simulink model "TST_EngDem_TrqLimCoord"  (R2016b)
settings: Solver=FixedStepDiscrete  StartTime=0.0  StopTime=0  FixedStep=sampleTime  RelTol=1e-3
values from neighbouring files (symbols this model uses):
  testCase = 1    [initTST_EngDem_TrqLimCoord_001.m]    (also in initTST_EngDem_TrqLimCoord_002.m = 2; initTST_EngDem_TrqLimCoord_003.m = 3; initTST_EngDem_TrqLimCoord_004.m = 4)
libraries: simulink x33, UnitTest_Lib x28
(part 1 of 2)
settings Model: Creator=zhengjinyan  LastModifiedBy=zhengjinyan
settings DebuggingCC: SignalRangeChecking=error

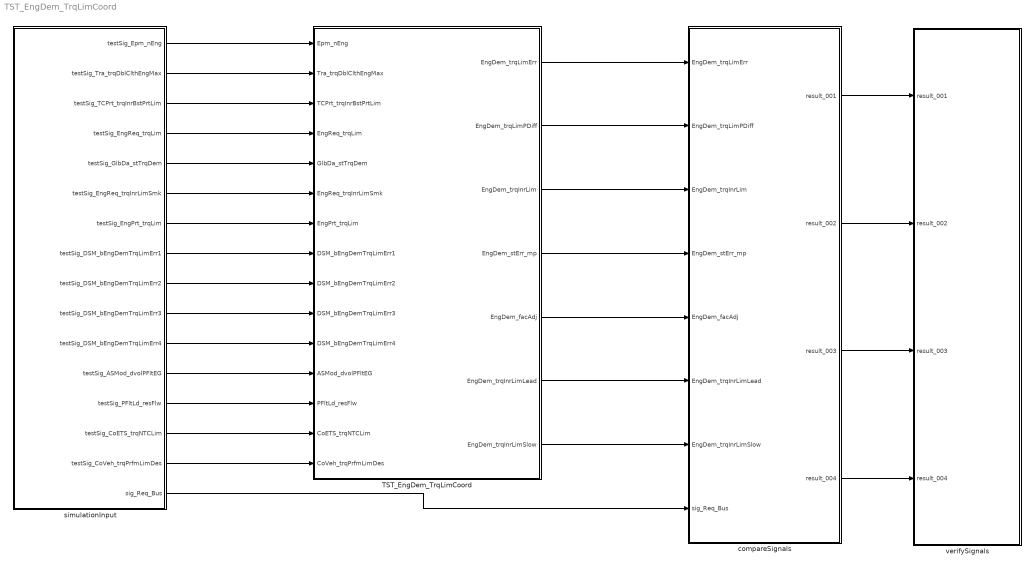
== system TST_EngDem_TrqLimCoord ==
  TST_EngDem_TrqLimCoord : Subsystem
  compareSignals : Subsystem
  simulationInput : Subsystem
  verifySignals : Subsystem
  wires:
  simulationInput/1(testSig_Epm_nEng) -> TST_EngDem_TrqLimCoord/1(Epm_nEng)
  simulationInput/2(testSig_Tra_trqDblClthEngMax) -> TST_EngDem_TrqLimCoord/2(Tra_trqDblClthEngMax)
  simulationInput/3(testSig_TCPrt_trqInrBstPrtLim) -> TST_EngDem_TrqLimCoord/3(TCPrt_trqInrBstPrtLim)
  simulationInput/4(testSig_EngReq_trqLim) -> TST_EngDem_TrqLimCoord/4(EngReq_trqLim)
  simulationInput/5(testSig_GlbDa_stTrqDem) -> TST_EngDem_TrqLimCoord/5(GlbDa_stTrqDem)
  simulationInput/6(testSig_EngReq_trqInrLimSmk) -> TST_EngDem_TrqLimCoord/6(EngReq_trqInrLimSmk)
  simulationInput/7(testSig_EngPrt_trqLim) -> TST_EngDem_TrqLimCoord/7(EngPrt_trqLim)
  simulationInput/8(testSig_DSM_bEngDemTrqLimErr1) -> TST_EngDem_TrqLimCoord/8(DSM_bEngDemTrqLimErr1)
  simulationInput/9(testSig_DSM_bEngDemTrqLimErr2) -> TST_EngDem_TrqLimCoord/9(DSM_bEngDemTrqLimErr2)
  simulationInput/10(testSig_DSM_bEngDemTrqLimErr3) -> TST_EngDem_TrqLimCoord/10(DSM_bEngDemTrqLimErr3)
  simulationInput/11(testSig_DSM_bEngDemTrqLimErr4) -> TST_EngDem_TrqLimCoord/11(DSM_bEngDemTrqLimErr4)
  simulationInput/12(testSig_ASMod_dvolPFltEG) -> TST_EngDem_TrqLimCoord/12(ASMod_dvolPFltEG)
  simulationInput/13(testSig_PFltLd_resFlw) -> TST_EngDem_TrqLimCoord/13(PFltLd_resFlw)
  simulationInput/14(testSig_CoETS_trqNTCLim) -> TST_EngDem_TrqLimCoord/14(CoETS_trqNTCLim)
  simulationInput/15(testSig_CoVeh_trqPrfmLimDes) -> TST_EngDem_TrqLimCoord/15(CoVeh_trqPrfmLimDes)
  TST_EngDem_TrqLimCoord/1(EngDem_trqLimErr) -> compareSignals/1(EngDem_trqLimErr)
  TST_EngDem_TrqLimCoord/2(EngDem_trqLimPDiff) -> compareSignals/2(EngDem_trqLimPDiff)
  TST_EngDem_TrqLimCoord/3(EngDem_trqInrLim) -> compareSignals/3(EngDem_trqInrLim)
  TST_EngDem_TrqLimCoord/4(EngDem_stErr_mp) -> compareSignals/4(EngDem_stErr_mp)
  TST_EngDem_TrqLimCoord/5(EngDem_facAdj) -> compareSignals/5(EngDem_facAdj)
  TST_EngDem_TrqLimCoord/6(EngDem_trqInrLimLead) -> compareSignals/6(EngDem_trqInrLimLead)
  TST_EngDem_TrqLimCoord/7(EngDem_trqInrLimSlow) -> compareSignals/7(EngDem_trqInrLimSlow)
  simulationInput/16(sig_Req_Bus) -> compareSignals/8(sig_Req_Bus)
  compareSignals/1(result_001) -> verifySignals/1(result_001)
  compareSignals/2(result_002) -> verifySignals/2(result_002)
  compareSignals/3(result_003) -> verifySignals/3(result_003)
  compareSignals/4(result_004) -> verifySignals/4(result_004)

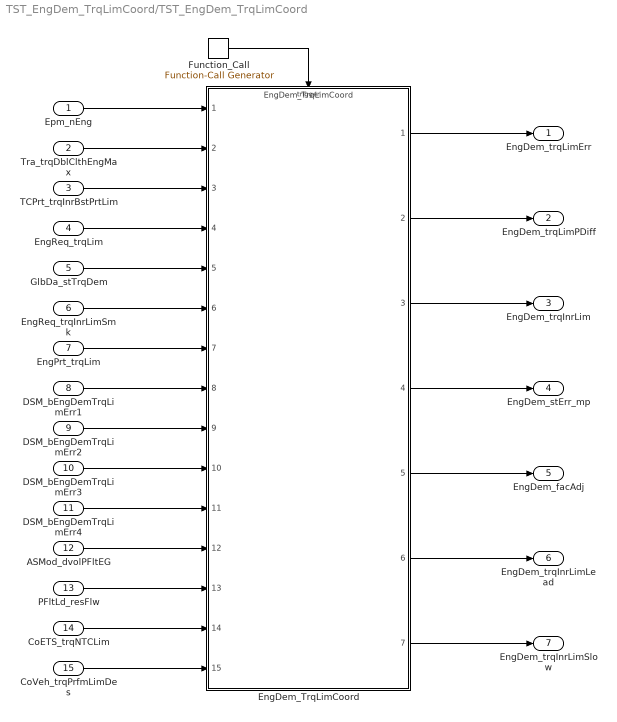
== system TST_EngDem_TrqLimCoord/TST_EngDem_TrqLimCoord ==
  Epm_nEng : Inport
  Tra_trqDblClthEngMax : Inport  Port=2
  TCPrt_trqInrBstPrtLim : Inport  Port=3
  EngReq_trqLim : Inport  Port=4
  GlbDa_stTrqDem : Inport  Port=5
  EngReq_trqInrLimSmk : Inport  Port=6
  EngPrt_trqLim : Inport  Port=7
  DSM_bEngDemTrqLimErr1 : Inport  Port=8
  DSM_bEngDemTrqLimErr2 : Inport  Port=9
  DSM_bEngDemTrqLimErr3 : Inport  Port=10
  DSM_bEngDemTrqLimErr4 : Inport  Port=11
  ASMod_dvolPFltEG : Inport  Port=12
  PFltLd_resFlw : Inport  Port=13
  CoETS_trqNTCLim : Inport  Port=14
  CoVeh_trqPrfmLimDes : Inport  Port=15
  EngDem_TrqLimCoord : ModelReference  ModelNameDialog=EngDem_TrqLimCoord  SimulationMode=Normal  ModelReferenceVersion=1.59  TriggerPortName=function  TriggerPortTriggerType=function-call  TriggerPortStatesWhenEnabling=held
  Function_Call : simulink/Ports & Subsystems/Function-Call Generator  sample_time=sampleTime  numberOfIterations=1
  EngDem_trqLimErr : Outport
  EngDem_trqLimPDiff : Outport  Port=2
  EngDem_trqInrLim : Outport  Port=3
  EngDem_stErr_mp : Outport  Port=4
  EngDem_facAdj : Outport  Port=5
  EngDem_trqInrLimLead : Outport  Port=6
  EngDem_trqInrLimSlow : Outport  Port=7
  wires:
  Function_Call/1 -> EngDem_TrqLimCoord/Trigger
  Epm_nEng/1 -> EngDem_TrqLimCoord/1
  Tra_trqDblClthEngMax/1 -> EngDem_TrqLimCoord/2
  TCPrt_trqInrBstPrtLim/1 -> EngDem_TrqLimCoord/3
  EngReq_trqLim/1 -> EngDem_TrqLimCoord/4
  GlbDa_stTrqDem/1 -> EngDem_TrqLimCoord/5
  EngReq_trqInrLimSmk/1 -> EngDem_TrqLimCoord/6
  EngPrt_trqLim/1 -> EngDem_TrqLimCoord/7
  DSM_bEngDemTrqLimErr1/1 -> EngDem_TrqLimCoord/8
  DSM_bEngDemTrqLimErr2/1 -> EngDem_TrqLimCoord/9
  DSM_bEngDemTrqLimErr3/1 -> EngDem_TrqLimCoord/10
  DSM_bEngDemTrqLimErr4/1 -> EngDem_TrqLimCoord/11
  ASMod_dvolPFltEG/1 -> EngDem_TrqLimCoord/12
  PFltLd_resFlw/1 -> EngDem_TrqLimCoord/13
  CoETS_trqNTCLim/1 -> EngDem_TrqLimCoord/14
  CoVeh_trqPrfmLimDes/1 -> EngDem_TrqLimCoord/15
  EngDem_TrqLimCoord/1 -> EngDem_trqLimErr/1
  EngDem_TrqLimCoord/2 -> EngDem_trqLimPDiff/1
  EngDem_TrqLimCoord/3 -> EngDem_trqInrLim/1
  EngDem_TrqLimCoord/4 -> EngDem_stErr_mp/1
  EngDem_TrqLimCoord/5 -> EngDem_facAdj/1
  EngDem_TrqLimCoord/6 -> EngDem_trqInrLimLead/1
  EngDem_TrqLimCoord/7 -> EngDem_trqInrLimSlow/1

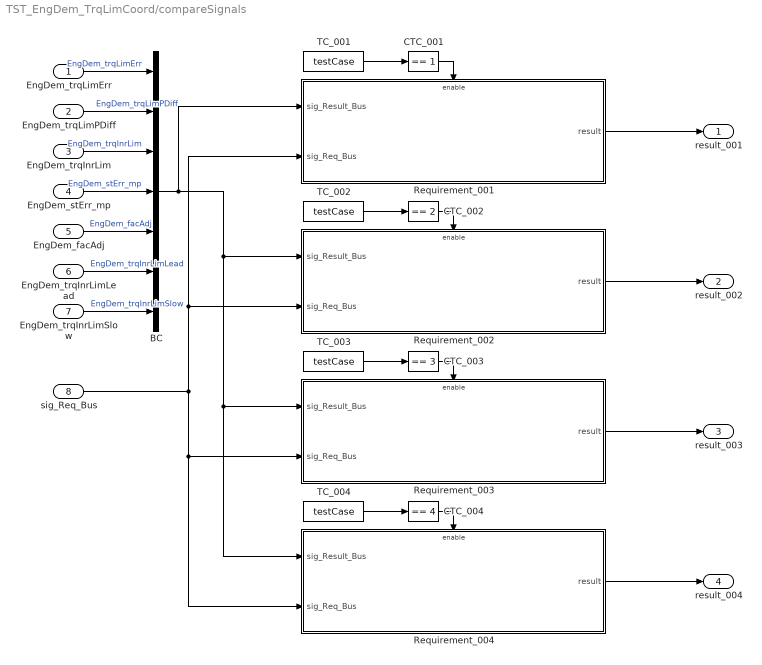
== system TST_EngDem_TrqLimCoord/compareSignals ==
  EngDem_trqLimErr : Inport
  EngDem_trqLimPDiff : Inport  Port=2
  EngDem_trqInrLim : Inport  Port=3
  EngDem_stErr_mp : Inport  Port=4
  EngDem_facAdj : Inport  Port=5
  EngDem_trqInrLimLead : Inport  Port=6
  EngDem_trqInrLimSlow : Inport  Port=7
  sig_Req_Bus : Inport  Port=8
  BC : BusCreator  Inputs=7
  CTC_001 : simulink/Logic and Bit Operations/Compare To Constant  relop===  const=1  OutDataTypeStr=boolean
  CTC_002 : simulink/Logic and Bit Operations/Compare To Constant  relop===  const=2  OutDataTypeStr=boolean
  CTC_003 : simulink/Logic and Bit Operations/Compare To Constant  relop===  const=3  OutDataTypeStr=boolean
  CTC_004 : simulink/Logic and Bit Operations/Compare To Constant  relop===  const=4  OutDataTypeStr=boolean
  Requirement_001 : Subsystem
  Requirement_002 : Subsystem
  Requirement_003 : Subsystem
  Requirement_004 : Subsystem
  TC_001 : Constant  Value=testCase
  TC_002 : Constant  Value=testCase
  TC_003 : Constant  Value=testCase
  TC_004 : Constant  Value=testCase
  result_001 : Outport
  result_002 : Outport  Port=2
  result_003 : Outport  Port=3
  result_004 : Outport  Port=4
  wires:
  EngDem_trqLimErr/1 -> BC/1  "EngDem_trqLimErr"
  EngDem_trqLimPDiff/1 -> BC/2  "EngDem_trqLimPDiff"
  EngDem_trqInrLim/1 -> BC/3  "EngDem_trqInrLim"
  EngDem_stErr_mp/1 -> BC/4  "EngDem_stErr_mp"
  EngDem_facAdj/1 -> BC/5  "EngDem_facAdj"
  EngDem_trqInrLimLead/1 -> BC/6  "EngDem_trqInrLimLead"
  EngDem_trqInrLimSlow/1 -> BC/7  "EngDem_trqInrLimSlow"
  TC_001/1 -> CTC_001/1
  CTC_001/1 -> Requirement_001/Enable
  sig_Req_Bus/1 -> Requirement_003/2(sig_Req_Bus), Requirement_004/2(sig_Req_Bus), Requirement_001/2(sig_Req_Bus), Requirement_002/2(sig_Req_Bus)
  BC/1 -> Requirement_003/1(sig_Result_Bus), Requirement_004/1(sig_Result_Bus), Requirement_002/1(sig_Result_Bus), Requirement_001/1(sig_Result_Bus)
  Requirement_001/1(result) -> result_001/1
  TC_002/1 -> CTC_002/1
  CTC_002/1 -> Requirement_002/Enable
  Requirement_002/1(result) -> result_002/1
  TC_003/1 -> CTC_003/1
  CTC_003/1 -> Requirement_003/Enable
  Requirement_003/1(result) -> result_003/1
  TC_004/1 -> CTC_004/1
  CTC_004/1 -> Requirement_004/Enable
  Requirement_004/1(result) -> result_004/1

== system TST_EngDem_TrqLimCoord/simulationInput ==
  BS : BusSelector  OutputSignals=testSig_Epm_nEng,testSig_Tra_trqDblClthEngMax,testSig_TCPrt_trqInrBstPrtLim,testSig_EngReq_trqLim,testSig_GlbDa_stTrqDem,testSig_EngReq_trqInrLimSmk,testSig_EngPrt_trqLim,testSig_DSM_bEngDemTrqLimErr1,testSig_DSM_bEngDemTrqLimErr2,testSig_DSM_bEngDemTrqLimErr3,testSig_DSM_bEngDemTrqLimErr4,testSig_ASMod_dvolPFltEG,testSig_PFltLd_resFlw,testSig_CoETS_trqNTCLim,testSig_CoVeh_trqPrfmLimDes
  MPSw : MultiPortSwitch  Inputs=4  SaturateOnIntegerOverflow=on  InputSameDT=on
  TestCase : Constant  Value=testCase
  testSignals_R001 : Subsystem
  testSignals_R002 : Subsystem
  testSignals_R003 : Subsystem
  testSignals_R004 : Subsystem
  testSig_Epm_nEng : Outport
  testSig_Tra_trqDblClthEngMax : Outport  Port=2
  testSig_TCPrt_trqInrBstPrtLim : Outport  Port=3
  testSig_EngReq_trqLim : Outport  Port=4
  testSig_GlbDa_stTrqDem : Outport  Port=5
  testSig_EngReq_trqInrLimSmk : Outport  Port=6
  testSig_EngPrt_trqLim : Outport  Port=7
  testSig_DSM_bEngDemTrqLimErr1 : Outport  Port=8
  testSig_DSM_bEngDemTrqLimErr2 : Outport  Port=9
  testSig_DSM_bEngDemTrqLimErr3 : Outport  Port=10
  testSig_DSM_bEngDemTrqLimErr4 : Outport  Port=11
  testSig_ASMod_dvolPFltEG : Outport  Port=12
  testSig_PFltLd_resFlw : Outport  Port=13
  testSig_CoETS_trqNTCLim : Outport  Port=14
  testSig_CoVeh_trqPrfmLimDes : Outport  Port=15
  sig_Req_Bus : Outport  Port=16
  wires:
  BS/1 -> testSig_Epm_nEng/1  "<testSig_Epm_nEng>"
  BS/2 -> testSig_Tra_trqDblClthEngMax/1  "<testSig_Tra_trqDblClthEngMax>"
  BS/3 -> testSig_TCPrt_trqInrBstPrtLim/1  "<testSig_TCPrt_trqInrBstPrtLim>"
  BS/4 -> testSig_EngReq_trqLim/1  "<testSig_EngReq_trqLim>"
  BS/5 -> testSig_GlbDa_stTrqDem/1  "<testSig_GlbDa_stTrqDem>"
  BS/6 -> testSig_EngReq_trqInrLimSmk/1  "<testSig_EngReq_trqInrLimSmk>"
  BS/7 -> testSig_EngPrt_trqLim/1  "<testSig_EngPrt_trqLim>"
  BS/8 -> testSig_DSM_bEngDemTrqLimErr1/1  "<testSig_DSM_bEngDemTrqLimErr1>"
  BS/9 -> testSig_DSM_bEngDemTrqLimErr2/1  "<testSig_DSM_bEngDemTrqLimErr2>"
  BS/10 -> testSig_DSM_bEngDemTrqLimErr3/1  "<testSig_DSM_bEngDemTrqLimErr3>"
  BS/11 -> testSig_DSM_bEngDemTrqLimErr4/1  "<testSig_DSM_bEngDemTrqLimErr4>"
  BS/12 -> testSig_ASMod_dvolPFltEG/1  "<testSig_ASMod_dvolPFltEG>"
  BS/13 -> testSig_PFltLd_resFlw/1  "<testSig_PFltLd_resFlw>"
  BS/14 -> testSig_CoETS_trqNTCLim/1  "<testSig_CoETS_trqNTCLim>"
  BS/15 -> testSig_CoVeh_trqPrfmLimDes/1  "<testSig_CoVeh_trqPrfmLimDes>"
  MPSw/1 -> BS/1, sig_Req_Bus/1
  TestCase/1 -> MPSw/1
  testSignals_R001/1(testSignals) -> MPSw/2
  testSignals_R002/1(testSignals) -> MPSw/3
  testSignals_R003/1(testSignals) -> MPSw/4
  testSignals_R004/1(testSignals) -> MPSw/5

== system TST_EngDem_TrqLimCoord/verifySignals ==
  result_001 : Inport
  result_002 : Inport  Port=2
  result_003 : Inport  Port=3
  result_004 : Inport  Port=4
  Assertion_001 : Assertion  Enabled=off
  Assertion_002 : Assertion  Enabled=off
  Assertion_003 : Assertion  Enabled=off
  Assertion_004 : Assertion  Enabled=off
  wires:
  result_001/1 -> Assertion_001/1
  result_002/1 -> Assertion_002/1
  result_003/1 -> Assertion_003/1
  result_004/1 -> Assertion_004/1

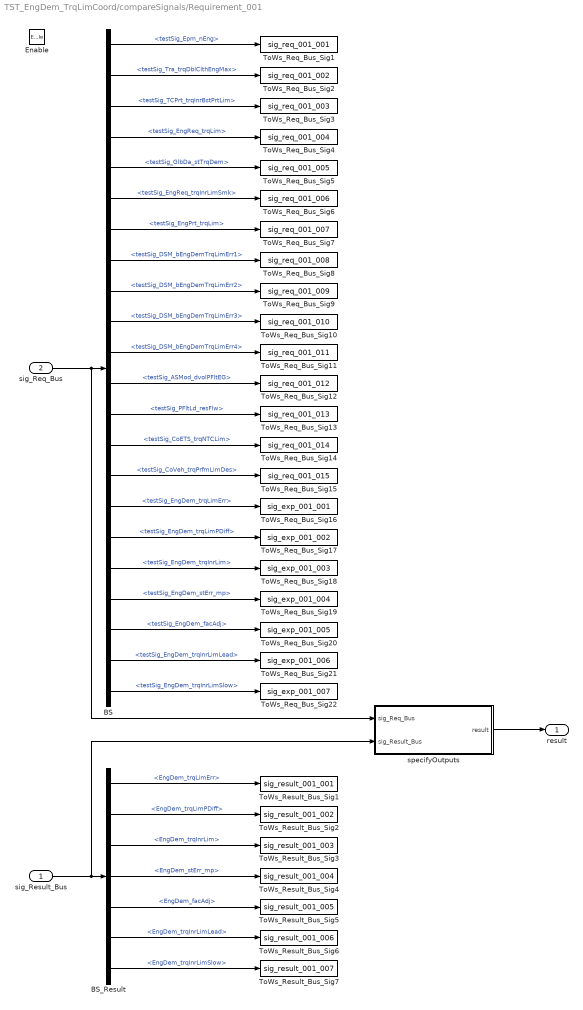
== system TST_EngDem_TrqLimCoord/compareSignals/Requirement_001 ==
  sig_Result_Bus : Inport
  sig_Req_Bus : Inport  Port=2
  Enable : EnablePort
  BS : BusSelector  OutputSignals=testSig_Epm_nEng,testSig_Tra_trqDblClthEngMax,testSig_TCPrt_trqInrBstPrtLim,testSig_EngReq_trqLim,testSig_GlbDa_stTrqDem,testSig_EngReq_trqInrLimSmk,testSig_EngPrt_trqLim,testSig_DSM_bEngDemTrqLimErr1,testSig_DSM_bEngDemTrqLimErr2,testSig_DSM_bEngDemTrqLimErr3,testSig_DSM_bEngDemTrqLimErr4,testSig_ASMod_dvolPFltEG,testSig_PFltLd_resFlw,testSig_CoETS_trqNTCLim,testSig_CoVeh_trqPrfmLimDes,testSig_EngDem_trqLimErr,testSig_EngDem_trqLimPDiff,testSig_EngDem_trqInrLim,testSig_EngDem_stErr_mp,testSig_EngDem_facAdj,testSig_EngDem_trqInrLimLead,testSig_EngDem_trqInrLimSlow
  BS_Result : BusSelector  OutputSignals=EngDem_trqLimErr,EngDem_trqLimPDiff,EngDem_trqInrLim,EngDem_stErr_mp,EngDem_facAdj,EngDem_trqInrLimLead,EngDem_trqInrLimSlow
  ToWs_Req_Bus_Sig1 : ToWorkspace  VariableName=sig_req_001_001  SaveFormat=Structure With Time
  ToWs_Req_Bus_Sig10 : ToWorkspace  VariableName=sig_req_001_010  SaveFormat=Structure With Time
  ToWs_Req_Bus_Sig11 : ToWorkspace  VariableName=sig_req_001_011  SaveFormat=Structure With Time
  ToWs_Req_Bus_Sig12 : ToWorkspace  VariableName=sig_req_001_012  SaveFormat=Structure With Time
  ToWs_Req_Bus_Sig13 : ToWorkspace  VariableName=sig_req_001_013  SaveFormat=Structure With Time
  ToWs_Req_Bus_Sig14 : ToWorkspace  VariableName=sig_req_001_014  SaveFormat=Structure With Time
  ToWs_Req_Bus_Sig15 : ToWorkspace  VariableName=sig_req_001_015  SaveFormat=Structure With Time
  ToWs_Req_Bus_Sig16 : ToWorkspace  VariableName=sig_exp_001_001  SaveFormat=Structure With Time
  ToWs_Req_Bus_Sig17 : ToWorkspace  VariableName=sig_exp_001_002  SaveFormat=Structure With Time
  ToWs_Req_Bus_Sig18 : ToWorkspace  VariableName=sig_exp_001_003  SaveFormat=Structure With Time
  ToWs_Req_Bus_Sig19 : ToWorkspace  VariableName=sig_exp_001_004  SaveFormat=Structure With Time
  ToWs_Req_Bus_Sig2 : ToWorkspace  VariableName=sig_req_001_002  SaveFormat=Structure With Time
  ToWs_Req_Bus_Sig20 : ToWorkspace  VariableName=sig_exp_001_005  SaveFormat=Structure With Time
  ToWs_Req_Bus_Sig21 : ToWorkspace  VariableName=sig_exp_001_006  SaveFormat=Structure With Time
  ToWs_Req_Bus_Sig22 : ToWorkspace  VariableName=sig_exp_001_007  SaveFormat=Structure With Time
  ToWs_Req_Bus_Sig3 : ToWorkspace  VariableName=sig_req_001_003  SaveFormat=Structure With Time
  ToWs_Req_Bus_Sig4 : ToWorkspace  VariableName=sig_req_001_004  SaveFormat=Structure With Time
  ToWs_Req_Bus_Sig5 : ToWorkspace  VariableName=sig_req_001_005  SaveFormat=Structure With Time
  ToWs_Req_Bus_Sig6 : ToWorkspace  VariableName=sig_req_001_006  SaveFormat=Structure With Time
  ToWs_Req_Bus_Sig7 : ToWorkspace  VariableName=sig_req_001_007  SaveFormat=Structure With Time
  ToWs_Req_Bus_Sig8 : ToWorkspace  VariableName=sig_req_001_008  SaveFormat=Structure With Time
  ToWs_Req_Bus_Sig9 : ToWorkspace  VariableName=sig_req_001_009  SaveFormat=Structure With Time
  ToWs_Result_Bus_Sig1 : ToWorkspace  VariableName=sig_result_001_001  SaveFormat=Structure With Time
  ToWs_Result_Bus_Sig2 : ToWorkspace  VariableName=sig_result_001_002  SaveFormat=Structure With Time
  ToWs_Result_Bus_Sig3 : ToWorkspace  VariableName=sig_result_001_003  SaveFormat=Structure With Time
  ToWs_Result_Bus_Sig4 : ToWorkspace  VariableName=sig_result_001_004  SaveFormat=Structure With Time
  ToWs_Result_Bus_Sig5 : ToWorkspace  VariableName=sig_result_001_005  SaveFormat=Structure With Time
  ToWs_Result_Bus_Sig6 : ToWorkspace  VariableName=sig_result_001_006  SaveFormat=Structure With Time
  ToWs_Result_Bus_Sig7 : ToWorkspace  VariableName=sig_result_001_007  SaveFormat=Structure With Time
  specifyOutputs : Subsystem
  result : Outport
  wires:
  sig_Req_Bus/1 -> BS/1, specifyOutputs/1(sig_Req_Bus)
  BS/1 -> ToWs_Req_Bus_Sig1/1  "<testSig_Epm_nEng>"
  BS/2 -> ToWs_Req_Bus_Sig2/1  "<testSig_Tra_trqDblClthEngMax>"
  BS/3 -> ToWs_Req_Bus_Sig3/1  "<testSig_TCPrt_trqInrBstPrtLim>"
  BS/4 -> ToWs_Req_Bus_Sig4/1  "<testSig_EngReq_trqLim>"
  BS/5 -> ToWs_Req_Bus_Sig5/1  "<testSig_GlbDa_stTrqDem>"
  BS/6 -> ToWs_Req_Bus_Sig6/1  "<testSig_EngReq_trqInrLimSmk>"
  BS/7 -> ToWs_Req_Bus_Sig7/1  "<testSig_EngPrt_trqLim>"
  BS/8 -> ToWs_Req_Bus_Sig8/1  "<testSig_DSM_bEngDemTrqLimErr1>"
  BS/9 -> ToWs_Req_Bus_Sig9/1  "<testSig_DSM_bEngDemTrqLimErr2>"
  BS/10 -> ToWs_Req_Bus_Sig10/1  "<testSig_DSM_bEngDemTrqLimErr3>"
  BS/11 -> ToWs_Req_Bus_Sig11/1  "<testSig_DSM_bEngDemTrqLimErr4>"
  BS/12 -> ToWs_Req_Bus_Sig12/1  "<testSig_ASMod_dvolPFltEG>"
  BS/13 -> ToWs_Req_Bus_Sig13/1  "<testSig_PFltLd_resFlw>"
  BS/14 -> ToWs_Req_Bus_Sig14/1  "<testSig_CoETS_trqNTCLim>"
  BS/15 -> ToWs_Req_Bus_Sig15/1  "<testSig_CoVeh_trqPrfmLimDes>"
  BS/16 -> ToWs_Req_Bus_Sig16/1  "<testSig_EngDem_trqLimErr>"
  BS/17 -> ToWs_Req_Bus_Sig17/1  "<testSig_EngDem_trqLimPDiff>"
  BS/18 -> ToWs_Req_Bus_Sig18/1  "<testSig_EngDem_trqInrLim>"
  BS/19 -> ToWs_Req_Bus_Sig19/1  "<testSig_EngDem_stErr_mp>"
  BS/20 -> ToWs_Req_Bus_Sig20/1  "<testSig_EngDem_facAdj>"
  BS/21 -> ToWs_Req_Bus_Sig21/1  "<testSig_EngDem_trqInrLimLead>"
  BS/22 -> ToWs_Req_Bus_Sig22/1  "<testSig_EngDem_trqInrLimSlow>"
  sig_Result_Bus/1 -> BS_Result/1, specifyOutputs/2(sig_Result_Bus)
  BS_Result/1 -> ToWs_Result_Bus_Sig1/1  "<EngDem_trqLimErr>"
  BS_Result/2 -> ToWs_Result_Bus_Sig2/1  "<EngDem_trqLimPDiff>"
  BS_Result/3 -> ToWs_Result_Bus_Sig3/1  "<EngDem_trqInrLim>"
  BS_Result/4 -> ToWs_Result_Bus_Sig4/1  "<EngDem_stErr_mp>"
  BS_Result/5 -> ToWs_Result_Bus_Sig5/1  "<EngDem_facAdj>"
  BS_Result/6 -> ToWs_Result_Bus_Sig6/1  "<EngDem_trqInrLimLead>"
  BS_Result/7 -> ToWs_Result_Bus_Sig7/1  "<EngDem_trqInrLimSlow>"
  specifyOutputs/1(result) -> result/1

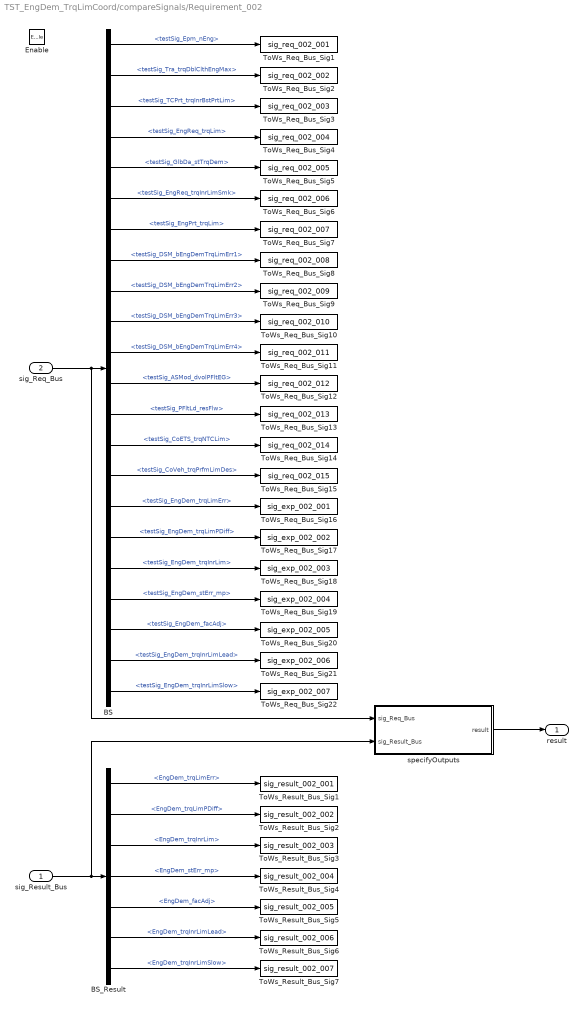
== system TST_EngDem_TrqLimCoord/compareSignals/Requirement_002 ==
  sig_Result_Bus : Inport
  sig_Req_Bus : Inport  Port=2
  Enable : EnablePort
  BS : BusSelector  OutputSignals=testSig_Epm_nEng,testSig_Tra_trqDblClthEngMax,testSig_TCPrt_trqInrBstPrtLim,testSig_EngReq_trqLim,testSig_GlbDa_stTrqDem,testSig_EngReq_trqInrLimSmk,testSig_EngPrt_trqLim,testSig_DSM_bEngDemTrqLimErr1,testSig_DSM_bEngDemTrqLimErr2,testSig_DSM_bEngDemTrqLimErr3,testSig_DSM_bEngDemTrqLimErr4,testSig_ASMod_dvolPFltEG,testSig_PFltLd_resFlw,testSig_CoETS_trqNTCLim,testSig_CoVeh_trqPrfmLimDes,testSig_EngDem_trqLimErr,testSig_EngDem_trqLimPDiff,testSig_EngDem_trqInrLim,testSig_EngDem_stErr_mp,testSig_EngDem_facAdj,testSig_EngDem_trqInrLimLead,testSig_EngDem_trqInrLimSlow
  BS_Result : BusSelector  OutputSignals=EngDem_trqLimErr,EngDem_trqLimPDiff,EngDem_trqInrLim,EngDem_stErr_mp,EngDem_facAdj,EngDem_trqInrLimLead,EngDem_trqInrLimSlow
  ToWs_Req_Bus_Sig1 : ToWorkspace  VariableName=sig_req_002_001  SaveFormat=Structure With Time
  ToWs_Req_Bus_Sig10 : ToWorkspace  VariableName=sig_req_002_010  SaveFormat=Structure With Time
  ToWs_Req_Bus_Sig11 : ToWorkspace  VariableName=sig_req_002_011  SaveFormat=Structure With Time
  ToWs_Req_Bus_Sig12 : ToWorkspace  VariableName=sig_req_002_012  SaveFormat=Structure With Time
  ToWs_Req_Bus_Sig13 : ToWorkspace  VariableName=sig_req_002_013  SaveFormat=Structure With Time
  ToWs_Req_Bus_Sig14 : ToWorkspace  VariableName=sig_req_002_014  SaveFormat=Structure With Time
  ToWs_Req_Bus_Sig15 : ToWorkspace  VariableName=sig_req_002_015  SaveFormat=Structure With Time
  ToWs_Req_Bus_Sig16 : ToWorkspace  VariableName=sig_exp_002_001  SaveFormat=Structure With Time
  ToWs_Req_Bus_Sig17 : ToWorkspace  VariableName=sig_exp_002_002  SaveFormat=Structure With Time
  ToWs_Req_Bus_Sig18 : ToWorkspace  VariableName=sig_exp_002_003  SaveFormat=Structure With Time
  ToWs_Req_Bus_Sig19 : ToWorkspace  VariableName=sig_exp_002_004  SaveFormat=Structure With Time
  ToWs_Req_Bus_Sig2 : ToWorkspace  VariableName=sig_req_002_002  SaveFormat=Structure With Time
  ToWs_Req_Bus_Sig20 : ToWorkspace  VariableName=sig_exp_002_005  SaveFormat=Structure With Time
  ToWs_Req_Bus_Sig21 : ToWorkspace  VariableName=sig_exp_002_006  SaveFormat=Structure With Time
  ToWs_Req_Bus_Sig22 : ToWorkspace  VariableName=sig_exp_002_007  SaveFormat=Structure With Time
  ToWs_Req_Bus_Sig3 : ToWorkspace  VariableName=sig_req_002_003  SaveFormat=Structure With Time
  ToWs_Req_Bus_Sig4 : ToWorkspace  VariableName=sig_req_002_004  SaveFormat=Structure With Time
  ToWs_Req_Bus_Sig5 : ToWorkspace  VariableName=sig_req_002_005  SaveFormat=Structure With Time
  ToWs_Req_Bus_Sig6 : ToWorkspace  VariableName=sig_req_002_006  SaveFormat=Structure With Time
  ToWs_Req_Bus_Sig7 : ToWorkspace  VariableName=sig_req_002_007  SaveFormat=Structure With Time
  ToWs_Req_Bus_Sig8 : ToWorkspace  VariableName=sig_req_002_008  SaveFormat=Structure With Time
  ToWs_Req_Bus_Sig9 : ToWorkspace  VariableName=sig_req_002_009  SaveFormat=Structure With Time
  ToWs_Result_Bus_Sig1 : ToWorkspace  VariableName=sig_result_002_001  SaveFormat=Structure With Time
  ToWs_Result_Bus_Sig2 : ToWorkspace  VariableName=sig_result_002_002  SaveFormat=Structure With Time
  ToWs_Result_Bus_Sig3 : ToWorkspace  VariableName=sig_result_002_003  SaveFormat=Structure With Time
  ToWs_Result_Bus_Sig4 : ToWorkspace  VariableName=sig_result_002_004  SaveFormat=Structure With Time
  ToWs_Result_Bus_Sig5 : ToWorkspace  VariableName=sig_result_002_005  SaveFormat=Structure With Time
  ToWs_Result_Bus_Sig6 : ToWorkspace  VariableName=sig_result_002_006  SaveFormat=Structure With Time
  ToWs_Result_Bus_Sig7 : ToWorkspace  VariableName=sig_result_002_007  SaveFormat=Structure With Time
  specifyOutputs : Subsystem
  result : Outport
  wires:
  sig_Req_Bus/1 -> BS/1, specifyOutputs/1(sig_Req_Bus)
  BS/1 -> ToWs_Req_Bus_Sig1/1  "<testSig_Epm_nEng>"
  BS/2 -> ToWs_Req_Bus_Sig2/1  "<testSig_Tra_trqDblClthEngMax>"
  BS/3 -> ToWs_Req_Bus_Sig3/1  "<testSig_TCPrt_trqInrBstPrtLim>"
  BS/4 -> ToWs_Req_Bus_Sig4/1  "<testSig_EngReq_trqLim>"
  BS/5 -> ToWs_Req_Bus_Sig5/1  "<testSig_GlbDa_stTrqDem>"
  BS/6 -> ToWs_Req_Bus_Sig6/1  "<testSig_EngReq_trqInrLimSmk>"
  BS/7 -> ToWs_Req_Bus_Sig7/1  "<testSig_EngPrt_trqLim>"
  BS/8 -> ToWs_Req_Bus_Sig8/1  "<testSig_DSM_bEngDemTrqLimErr1>"
  BS/9 -> ToWs_Req_Bus_Sig9/1  "<testSig_DSM_bEngDemTrqLimErr2>"
  BS/10 -> ToWs_Req_Bus_Sig10/1  "<testSig_DSM_bEngDemTrqLimErr3>"
  BS/11 -> ToWs_Req_Bus_Sig11/1  "<testSig_DSM_bEngDemTrqLimErr4>"
  BS/12 -> ToWs_Req_Bus_Sig12/1  "<testSig_ASMod_dvolPFltEG>"
  BS/13 -> ToWs_Req_Bus_Sig13/1  "<testSig_PFltLd_resFlw>"
  BS/14 -> ToWs_Req_Bus_Sig14/1  "<testSig_CoETS_trqNTCLim>"
  BS/15 -> ToWs_Req_Bus_Sig15/1  "<testSig_CoVeh_trqPrfmLimDes>"
  BS/16 -> ToWs_Req_Bus_Sig16/1  "<testSig_EngDem_trqLimErr>"
  BS/17 -> ToWs_Req_Bus_Sig17/1  "<testSig_EngDem_trqLimPDiff>"
  BS/18 -> ToWs_Req_Bus_Sig18/1  "<testSig_EngDem_trqInrLim>"
  BS/19 -> ToWs_Req_Bus_Sig19/1  "<testSig_EngDem_stErr_mp>"
  BS/20 -> ToWs_Req_Bus_Sig20/1  "<testSig_EngDem_facAdj>"
  BS/21 -> ToWs_Req_Bus_Sig21/1  "<testSig_EngDem_trqInrLimLead>"
  BS/22 -> ToWs_Req_Bus_Sig22/1  "<testSig_EngDem_trqInrLimSlow>"
  sig_Result_Bus/1 -> BS_Result/1, specifyOutputs/2(sig_Result_Bus)
  BS_Result/1 -> ToWs_Result_Bus_Sig1/1  "<EngDem_trqLimErr>"
  BS_Result/2 -> ToWs_Result_Bus_Sig2/1  "<EngDem_trqLimPDiff>"
  BS_Result/3 -> ToWs_Result_Bus_Sig3/1  "<EngDem_trqInrLim>"
  BS_Result/4 -> ToWs_Result_Bus_Sig4/1  "<EngDem_stErr_mp>"
  BS_Result/5 -> ToWs_Result_Bus_Sig5/1  "<EngDem_facAdj>"
  BS_Result/6 -> ToWs_Result_Bus_Sig6/1  "<EngDem_trqInrLimLead>"
  BS_Result/7 -> ToWs_Result_Bus_Sig7/1  "<EngDem_trqInrLimSlow>"
  specifyOutputs/1(result) -> result/1

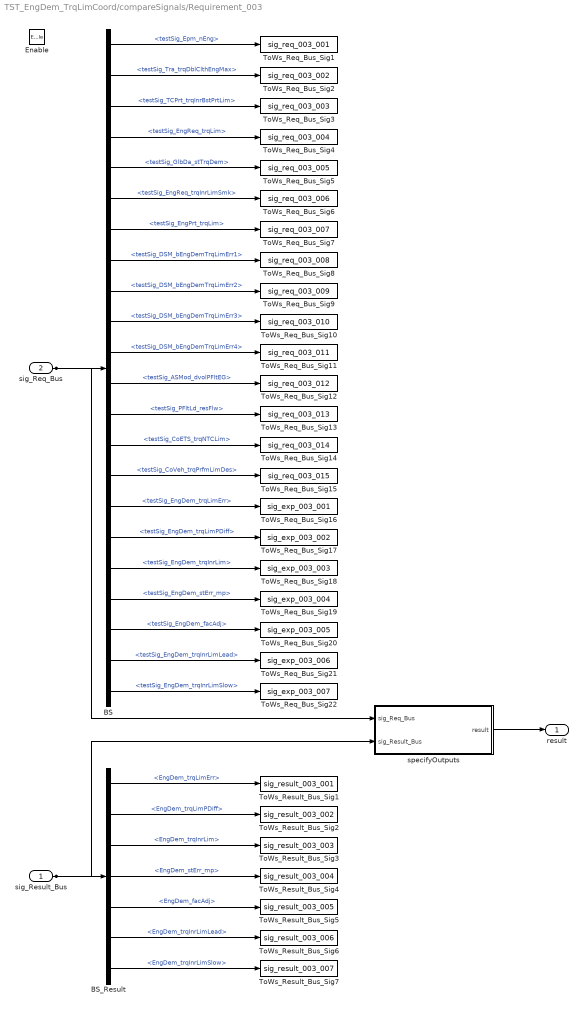
== system TST_EngDem_TrqLimCoord/compareSignals/Requirement_003 ==
  sig_Result_Bus : Inport
  sig_Req_Bus : Inport  Port=2
  Enable : EnablePort
  BS : BusSelector  OutputSignals=testSig_Epm_nEng,testSig_Tra_trqDblClthEngMax,testSig_TCPrt_trqInrBstPrtLim,testSig_EngReq_trqLim,testSig_GlbDa_stTrqDem,testSig_EngReq_trqInrLimSmk,testSig_EngPrt_trqLim,testSig_DSM_bEngDemTrqLimErr1,testSig_DSM_bEngDemTrqLimErr2,testSig_DSM_bEngDemTrqLimErr3,testSig_DSM_bEngDemTrqLimErr4,testSig_ASMod_dvolPFltEG,testSig_PFltLd_resFlw,testSig_CoETS_trqNTCLim,testSig_CoVeh_trqPrfmLimDes,testSig_EngDem_trqLimErr,testSig_EngDem_trqLimPDiff,testSig_EngDem_trqInrLim,testSig_EngDem_stErr_mp,testSig_EngDem_facAdj,testSig_EngDem_trqInrLimLead,testSig_EngDem_trqInrLimSlow
  BS_Result : BusSelector  OutputSignals=EngDem_trqLimErr,EngDem_trqLimPDiff,EngDem_trqInrLim,EngDem_stErr_mp,EngDem_facAdj,EngDem_trqInrLimLead,EngDem_trqInrLimSlow
  ToWs_Req_Bus_Sig1 : ToWorkspace  VariableName=sig_req_003_001  SaveFormat=Structure With Time
  ToWs_Req_Bus_Sig10 : ToWorkspace  VariableName=sig_req_003_010  SaveFormat=Structure With Time
  ToWs_Req_Bus_Sig11 : ToWorkspace  VariableName=sig_req_003_011  SaveFormat=Structure With Time
  ToWs_Req_Bus_Sig12 : ToWorkspace  VariableName=sig_req_003_012  SaveFormat=Structure With Time
  ToWs_Req_Bus_Sig13 : ToWorkspace  VariableName=sig_req_003_013  SaveFormat=Structure With Time
  ToWs_Req_Bus_Sig14 : ToWorkspace  VariableName=sig_req_003_014  SaveFormat=Structure With Time
  ToWs_Req_Bus_Sig15 : ToWorkspace  VariableName=sig_req_003_015  SaveFormat=Structure With Time
  ToWs_Req_Bus_Sig16 : ToWorkspace  VariableName=sig_exp_003_001  SaveFormat=Structure With Time
  ToWs_Req_Bus_Sig17 : ToWorkspace  VariableName=sig_exp_003_002  SaveFormat=Structure With Time
  ToWs_Req_Bus_Sig18 : ToWorkspace  VariableName=sig_exp_003_003  SaveFormat=Structure With Time
  ToWs_Req_Bus_Sig19 : ToWorkspace  VariableName=sig_exp_003_004  SaveFormat=Structure With Time
  ToWs_Req_Bus_Sig2 : ToWorkspace  VariableName=sig_req_003_002  SaveFormat=Structure With Time
  ToWs_Req_Bus_Sig20 : ToWorkspace  VariableName=sig_exp_003_005  SaveFormat=Structure With Time
  ToWs_Req_Bus_Sig21 : ToWorkspace  VariableName=sig_exp_003_006  SaveFormat=Structure With Time
  ToWs_Req_Bus_Sig22 : ToWorkspace  VariableName=sig_exp_003_007  SaveFormat=Structure With Time
  ToWs_Req_Bus_Sig3 : ToWorkspace  VariableName=sig_req_003_003  SaveFormat=Structure With Time
  ToWs_Req_Bus_Sig4 : ToWorkspace  VariableName=sig_req_003_004  SaveFormat=Structure With Time
  ToWs_Req_Bus_Sig5 : ToWorkspace  VariableName=sig_req_003_005  SaveFormat=Structure With Time
  ToWs_Req_Bus_Sig6 : ToWorkspace  VariableName=sig_req_003_006  SaveFormat=Structure With Time
  ToWs_Req_Bus_Sig7 : ToWorkspace  VariableName=sig_req_003_007  SaveFormat=Structure With Time
  ToWs_Req_Bus_Sig8 : ToWorkspace  VariableName=sig_req_003_008  SaveFormat=Structure With Time
  ToWs_Req_Bus_Sig9 : ToWorkspace  VariableName=sig_req_003_009  SaveFormat=Structure With Time
  ToWs_Result_Bus_Sig1 : ToWorkspace  VariableName=sig_result_003_001  SaveFormat=Structure With Time
  ToWs_Result_Bus_Sig2 : ToWorkspace  VariableName=sig_result_003_002  SaveFormat=Structure With Time
  ToWs_Result_Bus_Sig3 : ToWorkspace  VariableName=sig_result_003_003  SaveFormat=Structure With Time
  ToWs_Result_Bus_Sig4 : ToWorkspace  VariableName=sig_result_003_004  SaveFormat=Structure With Time
  ToWs_Result_Bus_Sig5 : ToWorkspace  VariableName=sig_result_003_005  SaveFormat=Structure With Time
  ToWs_Result_Bus_Sig6 : ToWorkspace  VariableName=sig_result_003_006  SaveFormat=Structure With Time
  ToWs_Result_Bus_Sig7 : ToWorkspace  VariableName=sig_result_003_007  SaveFormat=Structure With Time
  specifyOutputs : Subsystem
  result : Outport
  wires:
  sig_Req_Bus/1 -> BS/1, specifyOutputs/1(sig_Req_Bus)
  BS/1 -> ToWs_Req_Bus_Sig1/1  "<testSig_Epm_nEng>"
  BS/2 -> ToWs_Req_Bus_Sig2/1  "<testSig_Tra_trqDblClthEngMax>"
  BS/3 -> ToWs_Req_Bus_Sig3/1  "<testSig_TCPrt_trqInrBstPrtLim>"
  BS/4 -> ToWs_Req_Bus_Sig4/1  "<testSig_EngReq_trqLim>"
  BS/5 -> ToWs_Req_Bus_Sig5/1  "<testSig_GlbDa_stTrqDem>"
  BS/6 -> ToWs_Req_Bus_Sig6/1  "<testSig_EngReq_trqInrLimSmk>"
  BS/7 -> ToWs_Req_Bus_Sig7/1  "<testSig_EngPrt_trqLim>"
  BS/8 -> ToWs_Req_Bus_Sig8/1  "<testSig_DSM_bEngDemTrqLimErr1>"
  BS/9 -> ToWs_Req_Bus_Sig9/1  "<testSig_DSM_bEngDemTrqLimErr2>"
  BS/10 -> ToWs_Req_Bus_Sig10/1  "<testSig_DSM_bEngDemTrqLimErr3>"
  BS/11 -> ToWs_Req_Bus_Sig11/1  "<testSig_DSM_bEngDemTrqLimErr4>"
  BS/12 -> ToWs_Req_Bus_Sig12/1  "<testSig_ASMod_dvolPFltEG>"
  BS/13 -> ToWs_Req_Bus_Sig13/1  "<testSig_PFltLd_resFlw>"
  BS/14 -> ToWs_Req_Bus_Sig14/1  "<testSig_CoETS_trqNTCLim>"
  BS/15 -> ToWs_Req_Bus_Sig15/1  "<testSig_CoVeh_trqPrfmLimDes>"
  BS/16 -> ToWs_Req_Bus_Sig16/1  "<testSig_EngDem_trqLimErr>"
  BS/17 -> ToWs_Req_Bus_Sig17/1  "<testSig_EngDem_trqLimPDiff>"
  BS/18 -> ToWs_Req_Bus_Sig18/1  "<testSig_EngDem_trqInrLim>"
  BS/19 -> ToWs_Req_Bus_Sig19/1  "<testSig_EngDem_stErr_mp>"
  BS/20 -> ToWs_Req_Bus_Sig20/1  "<testSig_EngDem_facAdj>"
  BS/21 -> ToWs_Req_Bus_Sig21/1  "<testSig_EngDem_trqInrLimLead>"
  BS/22 -> ToWs_Req_Bus_Sig22/1  "<testSig_EngDem_trqInrLimSlow>"
  sig_Result_Bus/1 -> BS_Result/1, specifyOutputs/2(sig_Result_Bus)
  BS_Result/1 -> ToWs_Result_Bus_Sig1/1  "<EngDem_trqLimErr>"
  BS_Result/2 -> ToWs_Result_Bus_Sig2/1  "<EngDem_trqLimPDiff>"
  BS_Result/3 -> ToWs_Result_Bus_Sig3/1  "<EngDem_trqInrLim>"
  BS_Result/4 -> ToWs_Result_Bus_Sig4/1  "<EngDem_stErr_mp>"
  BS_Result/5 -> ToWs_Result_Bus_Sig5/1  "<EngDem_facAdj>"
  BS_Result/6 -> ToWs_Result_Bus_Sig6/1  "<EngDem_trqInrLimLead>"
  BS_Result/7 -> ToWs_Result_Bus_Sig7/1  "<EngDem_trqInrLimSlow>"
  specifyOutputs/1(result) -> result/1

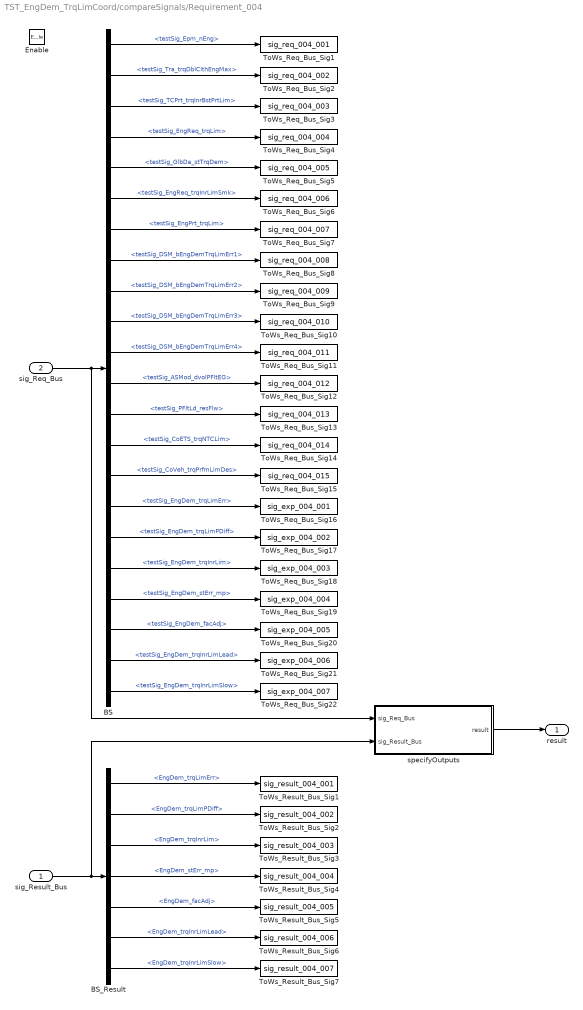
== system TST_EngDem_TrqLimCoord/compareSignals/Requirement_004 ==
  sig_Result_Bus : Inport
  sig_Req_Bus : Inport  Port=2
  Enable : EnablePort
  BS : BusSelector  OutputSignals=testSig_Epm_nEng,testSig_Tra_trqDblClthEngMax,testSig_TCPrt_trqInrBstPrtLim,testSig_EngReq_trqLim,testSig_GlbDa_stTrqDem,testSig_EngReq_trqInrLimSmk,testSig_EngPrt_trqLim,testSig_DSM_bEngDemTrqLimErr1,testSig_DSM_bEngDemTrqLimErr2,testSig_DSM_bEngDemTrqLimErr3,testSig_DSM_bEngDemTrqLimErr4,testSig_ASMod_dvolPFltEG,testSig_PFltLd_resFlw,testSig_CoETS_trqNTCLim,testSig_CoVeh_trqPrfmLimDes,testSig_EngDem_trqLimErr,testSig_EngDem_trqLimPDiff,testSig_EngDem_trqInrLim,testSig_EngDem_stErr_mp,testSig_EngDem_facAdj,testSig_EngDem_trqInrLimLead,testSig_EngDem_trqInrLimSlow
  BS_Result : BusSelector  OutputSignals=EngDem_trqLimErr,EngDem_trqLimPDiff,EngDem_trqInrLim,EngDem_stErr_mp,EngDem_facAdj,EngDem_trqInrLimLead,EngDem_trqInrLimSlow
  ToWs_Req_Bus_Sig1 : ToWorkspace  VariableName=sig_req_004_001  SaveFormat=Structure With Time
  ToWs_Req_Bus_Sig10 : ToWorkspace  VariableName=sig_req_004_010  SaveFormat=Structure With Time
  ToWs_Req_Bus_Sig11 : ToWorkspace  VariableName=sig_req_004_011  SaveFormat=Structure With Time
  ToWs_Req_Bus_Sig12 : ToWorkspace  VariableName=sig_req_004_012  SaveFormat=Structure With Time
  ToWs_Req_Bus_Sig13 : ToWorkspace  VariableName=sig_req_004_013  SaveFormat=Structure With Time
  ToWs_Req_Bus_Sig14 : ToWorkspace  VariableName=sig_req_004_014  SaveFormat=Structure With Time
  ToWs_Req_Bus_Sig15 : ToWorkspace  VariableName=sig_req_004_015  SaveFormat=Structure With Time
  ToWs_Req_Bus_Sig16 : ToWorkspace  VariableName=sig_exp_004_001  SaveFormat=Structure With Time
  ToWs_Req_Bus_Sig17 : ToWorkspace  VariableName=sig_exp_004_002  SaveFormat=Structure With Time
  ToWs_Req_Bus_Sig18 : ToWorkspace  VariableName=sig_exp_004_003  SaveFormat=Structure With Time
  ToWs_Req_Bus_Sig19 : ToWorkspace  VariableName=sig_exp_004_004  SaveFormat=Structure With Time
  ToWs_Req_Bus_Sig2 : ToWorkspace  VariableName=sig_req_004_002  SaveFormat=Structure With Time
  ToWs_Req_Bus_Sig20 : ToWorkspace  VariableName=sig_exp_004_005  SaveFormat=Structure With Time
  ToWs_Req_Bus_Sig21 : ToWorkspace  VariableName=sig_exp_004_006  SaveFormat=Structure With Time
  ToWs_Req_Bus_Sig22 : ToWorkspace  VariableName=sig_exp_004_007  SaveFormat=Structure With Time
  ToWs_Req_Bus_Sig3 : ToWorkspace  VariableName=sig_req_004_003  SaveFormat=Structure With Time
  ToWs_Req_Bus_Sig4 : ToWorkspace  VariableName=sig_req_004_004  SaveFormat=Structure With Time
  ToWs_Req_Bus_Sig5 : ToWorkspace  VariableName=sig_req_004_005  SaveFormat=Structure With Time
  ToWs_Req_Bus_Sig6 : ToWorkspace  VariableName=sig_req_004_006  SaveFormat=Structure With Time
  ToWs_Req_Bus_Sig7 : ToWorkspace  VariableName=sig_req_004_007  SaveFormat=Structure With Time
  ToWs_Req_Bus_Sig8 : ToWorkspace  VariableName=sig_req_004_008  SaveFormat=Structure With Time
  ToWs_Req_Bus_Sig9 : ToWorkspace  VariableName=sig_req_004_009  SaveFormat=Structure With Time
  ToWs_Result_Bus_Sig1 : ToWorkspace  VariableName=sig_result_004_001  SaveFormat=Structure With Time
  ToWs_Result_Bus_Sig2 : ToWorkspace  VariableName=sig_result_004_002  SaveFormat=Structure With Time
  ToWs_Result_Bus_Sig3 : ToWorkspace  VariableName=sig_result_004_003  SaveFormat=Structure With Time
  ToWs_Result_Bus_Sig4 : ToWorkspace  VariableName=sig_result_004_004  SaveFormat=Structure With Time
  ToWs_Result_Bus_Sig5 : ToWorkspace  VariableName=sig_result_004_005  SaveFormat=Structure With Time
  ToWs_Result_Bus_Sig6 : ToWorkspace  VariableName=sig_result_004_006  SaveFormat=Structure With Time
  ToWs_Result_Bus_Sig7 : ToWorkspace  VariableName=sig_result_004_007  SaveFormat=Structure With Time
  specifyOutputs : Subsystem
  result : Outport
  wires:
  sig_Req_Bus/1 -> BS/1, specifyOutputs/1(sig_Req_Bus)
  BS/1 -> ToWs_Req_Bus_Sig1/1  "<testSig_Epm_nEng>"
  BS/2 -> ToWs_Req_Bus_Sig2/1  "<testSig_Tra_trqDblClthEngMax>"
  BS/3 -> ToWs_Req_Bus_Sig3/1  "<testSig_TCPrt_trqInrBstPrtLim>"
  BS/4 -> ToWs_Req_Bus_Sig4/1  "<testSig_EngReq_trqLim>"
  BS/5 -> ToWs_Req_Bus_Sig5/1  "<testSig_GlbDa_stTrqDem>"
  BS/6 -> ToWs_Req_Bus_Sig6/1  "<testSig_EngReq_trqInrLimSmk>"
  BS/7 -> ToWs_Req_Bus_Sig7/1  "<testSig_EngPrt_trqLim>"
  BS/8 -> ToWs_Req_Bus_Sig8/1  "<testSig_DSM_bEngDemTrqLimErr1>"
  BS/9 -> ToWs_Req_Bus_Sig9/1  "<testSig_DSM_bEngDemTrqLimErr2>"
  BS/10 -> ToWs_Req_Bus_Sig10/1  "<testSig_DSM_bEngDemTrqLimErr3>"
  BS/11 -> ToWs_Req_Bus_Sig11/1  "<testSig_DSM_bEngDemTrqLimErr4>"
  BS/12 -> ToWs_Req_Bus_Sig12/1  "<testSig_ASMod_dvolPFltEG>"
  BS/13 -> ToWs_Req_Bus_Sig13/1  "<testSig_PFltLd_resFlw>"
  BS/14 -> ToWs_Req_Bus_Sig14/1  "<testSig_CoETS_trqNTCLim>"
  BS/15 -> ToWs_Req_Bus_Sig15/1  "<testSig_CoVeh_trqPrfmLimDes>"
  BS/16 -> ToWs_Req_Bus_Sig16/1  "<testSig_EngDem_trqLimErr>"
  BS/17 -> ToWs_Req_Bus_Sig17/1  "<testSig_EngDem_trqLimPDiff>"
  BS/18 -> ToWs_Req_Bus_Sig18/1  "<testSig_EngDem_trqInrLim>"
  BS/19 -> ToWs_Req_Bus_Sig19/1  "<testSig_EngDem_stErr_mp>"
  BS/20 -> ToWs_Req_Bus_Sig20/1  "<testSig_EngDem_facAdj>"
  BS/21 -> ToWs_Req_Bus_Sig21/1  "<testSig_EngDem_trqInrLimLead>"
  BS/22 -> ToWs_Req_Bus_Sig22/1  "<testSig_EngDem_trqInrLimSlow>"
  sig_Result_Bus/1 -> BS_Result/1, specifyOutputs/2(sig_Result_Bus)
  BS_Result/1 -> ToWs_Result_Bus_Sig1/1  "<EngDem_trqLimErr>"
  BS_Result/2 -> ToWs_Result_Bus_Sig2/1  "<EngDem_trqLimPDiff>"
  BS_Result/3 -> ToWs_Result_Bus_Sig3/1  "<EngDem_trqInrLim>"
  BS_Result/4 -> ToWs_Result_Bus_Sig4/1  "<EngDem_stErr_mp>"
  BS_Result/5 -> ToWs_Result_Bus_Sig5/1  "<EngDem_facAdj>"
  BS_Result/6 -> ToWs_Result_Bus_Sig6/1  "<EngDem_trqInrLimLead>"
  BS_Result/7 -> ToWs_Result_Bus_Sig7/1  "<EngDem_trqInrLimSlow>"
  specifyOutputs/1(result) -> result/1

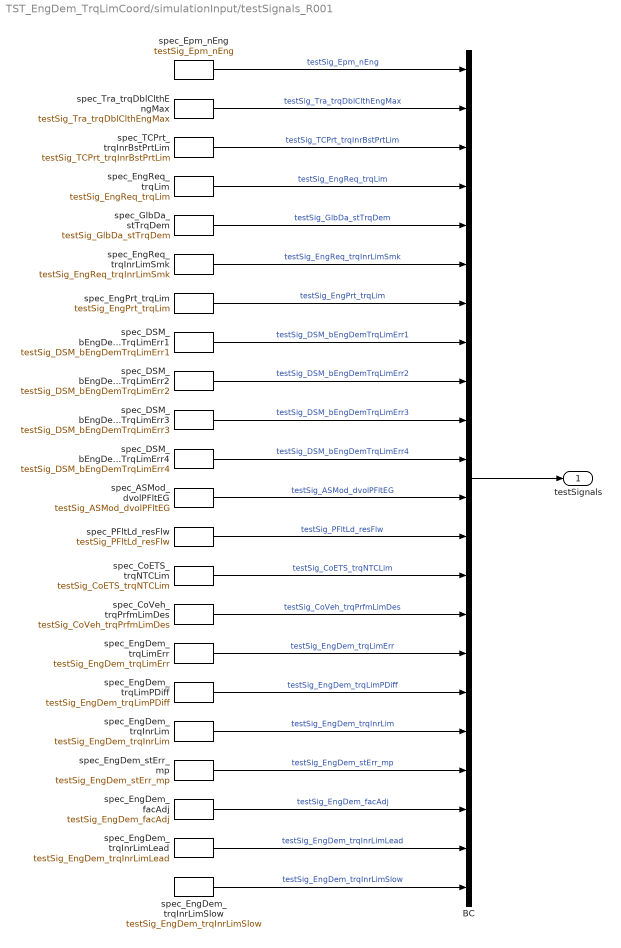
== system TST_EngDem_TrqLimCoord/simulationInput/testSignals_R001 ==
  BC : BusCreator  Inputs=22
  spec_ASMod_dvolPFltEG : FromWorkspace  VariableName=testSig_ASMod_dvolPFltEG  Interpolate=off  OutputAfterFinalValue=Holding final value
  spec_CoETS_trqNTCLim : FromWorkspace  VariableName=testSig_CoETS_trqNTCLim  Interpolate=off  OutputAfterFinalValue=Holding final value
  spec_CoVeh_trqPrfmLimDes : FromWorkspace  VariableName=testSig_CoVeh_trqPrfmLimDes  Interpolate=off  OutputAfterFinalValue=Holding final value
  spec_DSM_bEngDemTrqLimErr1 : FromWorkspace  VariableName=testSig_DSM_bEngDemTrqLimErr1  Interpolate=off  OutputAfterFinalValue=Holding final value
  spec_DSM_bEngDemTrqLimErr2 : FromWorkspace  VariableName=testSig_DSM_bEngDemTrqLimErr2  Interpolate=off  OutputAfterFinalValue=Holding final value
  spec_DSM_bEngDemTrqLimErr3 : FromWorkspace  VariableName=testSig_DSM_bEngDemTrqLimErr3  Interpolate=off  OutputAfterFinalValue=Holding final value
  spec_DSM_bEngDemTrqLimErr4 : FromWorkspace  VariableName=testSig_DSM_bEngDemTrqLimErr4  Interpolate=off  OutputAfterFinalValue=Holding final value
  spec_EngDem_facAdj : FromWorkspace  VariableName=testSig_EngDem_facAdj  Interpolate=off  OutputAfterFinalValue=Holding final value
  spec_EngDem_stErr_mp : FromWorkspace  VariableName=testSig_EngDem_stErr_mp  Interpolate=off  OutputAfterFinalValue=Holding final value
  spec_EngDem_trqInrLim : FromWorkspace  VariableName=testSig_EngDem_trqInrLim  Interpolate=off  OutputAfterFinalValue=Holding final value
  spec_EngDem_trqInrLimLead : FromWorkspace  VariableName=testSig_EngDem_trqInrLimLead  Interpolate=off  OutputAfterFinalValue=Holding final value
  spec_EngDem_trqInrLimSlow : FromWorkspace  VariableName=testSig_EngDem_trqInrLimSlow  Interpolate=off  OutputAfterFinalValue=Holding final value
  spec_EngDem_trqLimErr : FromWorkspace  VariableName=testSig_EngDem_trqLimErr  Interpolate=off  OutputAfterFinalValue=Holding final value
  spec_EngDem_trqLimPDiff : FromWorkspace  VariableName=testSig_EngDem_trqLimPDiff  Interpolate=off  OutputAfterFinalValue=Holding final value
  spec_EngPrt_trqLim : FromWorkspace  VariableName=testSig_EngPrt_trqLim  Interpolate=off  OutputAfterFinalValue=Holding final value
  spec_EngReq_trqInrLimSmk : FromWorkspace  VariableName=testSig_EngReq_trqInrLimSmk  Interpolate=off  OutputAfterFinalValue=Holding final value
  spec_EngReq_trqLim : FromWorkspace  VariableName=testSig_EngReq_trqLim  Interpolate=off  OutputAfterFinalValue=Holding final value
  spec_Epm_nEng : FromWorkspace  VariableName=testSig_Epm_nEng  Interpolate=off  OutputAfterFinalValue=Holding final value
  spec_GlbDa_stTrqDem : FromWorkspace  VariableName=testSig_GlbDa_stTrqDem  Interpolate=off  OutputAfterFinalValue=Holding final value
  spec_PFltLd_resFlw : FromWorkspace  VariableName=testSig_PFltLd_resFlw  Interpolate=off  OutputAfterFinalValue=Holding final value
  spec_TCPrt_trqInrBstPrtLim : FromWorkspace  VariableName=testSig_TCPrt_trqInrBstPrtLim  Interpolate=off  OutputAfterFinalValue=Holding final value
  spec_Tra_trqDblClthEngMax : FromWorkspace  VariableName=testSig_Tra_trqDblClthEngMax  Interpolate=off  OutputAfterFinalValue=Holding final value
  testSignals : Outport
  wires:
  BC/1 -> testSignals/1
  spec_Epm_nEng/1 -> BC/1  "testSig_Epm_nEng"
  spec_Tra_trqDblClthEngMax/1 -> BC/2  "testSig_Tra_trqDblClthEngMax"
  spec_TCPrt_trqInrBstPrtLim/1 -> BC/3  "testSig_TCPrt_trqInrBstPrtLim"
  spec_EngReq_trqLim/1 -> BC/4  "testSig_EngReq_trqLim"
  spec_GlbDa_stTrqDem/1 -> BC/5  "testSig_GlbDa_stTrqDem"
  spec_EngReq_trqInrLimSmk/1 -> BC/6  "testSig_EngReq_trqInrLimSmk"
  spec_EngPrt_trqLim/1 -> BC/7  "testSig_EngPrt_trqLim"
  spec_DSM_bEngDemTrqLimErr1/1 -> BC/8  "testSig_DSM_bEngDemTrqLimErr1"
  spec_DSM_bEngDemTrqLimErr2/1 -> BC/9  "testSig_DSM_bEngDemTrqLimErr2"
  spec_DSM_bEngDemTrqLimErr3/1 -> BC/10  "testSig_DSM_bEngDemTrqLimErr3"
  spec_DSM_bEngDemTrqLimErr4/1 -> BC/11  "testSig_DSM_bEngDemTrqLimErr4"
  spec_ASMod_dvolPFltEG/1 -> BC/12  "testSig_ASMod_dvolPFltEG"
  spec_PFltLd_resFlw/1 -> BC/13  "testSig_PFltLd_resFlw"
  spec_CoETS_trqNTCLim/1 -> BC/14  "testSig_CoETS_trqNTCLim"
  spec_CoVeh_trqPrfmLimDes/1 -> BC/15  "testSig_CoVeh_trqPrfmLimDes"
  spec_EngDem_trqLimErr/1 -> BC/16  "testSig_EngDem_trqLimErr"
  spec_EngDem_trqLimPDiff/1 -> BC/17  "testSig_EngDem_trqLimPDiff"
  spec_EngDem_trqInrLim/1 -> BC/18  "testSig_EngDem_trqInrLim"
  spec_EngDem_stErr_mp/1 -> BC/19  "testSig_EngDem_stErr_mp"
  spec_EngDem_facAdj/1 -> BC/20  "testSig_EngDem_facAdj"
  spec_EngDem_trqInrLimLead/1 -> BC/21  "testSig_EngDem_trqInrLimLead"
  spec_EngDem_trqInrLimSlow/1 -> BC/22  "testSig_EngDem_trqInrLimSlow"

== system TST_EngDem_TrqLimCoord/simulationInput/testSignals_R002 ==
  BC : BusCreator  Inputs=22
  spec_ASMod_dvolPFltEG : FromWorkspace  VariableName=testSig_ASMod_dvolPFltEG  Interpolate=off  OutputAfterFinalValue=Holding final value
  spec_CoETS_trqNTCLim : FromWorkspace  VariableName=testSig_CoETS_trqNTCLim  Interpolate=off  OutputAfterFinalValue=Holding final value
  spec_CoVeh_trqPrfmLimDes : FromWorkspace  VariableName=testSig_CoVeh_trqPrfmLimDes  Interpolate=off  OutputAfterFinalValue=Holding final value
  spec_DSM_bEngDemTrqLimErr1 : FromWorkspace  VariableName=testSig_DSM_bEngDemTrqLimErr1  Interpolate=off  OutputAfterFinalValue=Holding final value
  spec_DSM_bEngDemTrqLimErr2 : FromWorkspace  VariableName=testSig_DSM_bEngDemTrqLimErr2  Interpolate=off  OutputAfterFinalValue=Holding final value
  spec_DSM_bEngDemTrqLimErr3 : FromWorkspace  VariableName=testSig_DSM_bEngDemTrqLimErr3  Interpolate=off  OutputAfterFinalValue=Holding final value
  spec_DSM_bEngDemTrqLimErr4 : FromWorkspace  VariableName=testSig_DSM_bEngDemTrqLimErr4  Interpolate=off  OutputAfterFinalValue=Holding final value
  spec_EngDem_facAdj : FromWorkspace  VariableName=testSig_EngDem_facAdj  Interpolate=off  OutputAfterFinalValue=Holding final value
  spec_EngDem_stErr_mp : FromWorkspace  VariableName=testSig_EngDem_stErr_mp  Interpolate=off  OutputAfterFinalValue=Holding final value
  spec_EngDem_trqInrLim : FromWorkspace  VariableName=testSig_EngDem_trqInrLim  Interpolate=off  OutputAfterFinalValue=Holding final value
  spec_EngDem_trqInrLimLead : FromWorkspace  VariableName=testSig_EngDem_trqInrLimLead  Interpolate=off  OutputAfterFinalValue=Holding final value
  spec_EngDem_trqInrLimSlow : FromWorkspace  VariableName=testSig_EngDem_trqInrLimSlow  Interpolate=off  OutputAfterFinalValue=Holding final value
  spec_EngDem_trqLimErr : FromWorkspace  VariableName=testSig_EngDem_trqLimErr  Interpolate=off  OutputAfterFinalValue=Holding final value
  spec_EngDem_trqLimPDiff : FromWorkspace  VariableName=testSig_EngDem_trqLimPDiff  Interpolate=off  OutputAfterFinalValue=Holding final value
  spec_EngPrt_trqLim : FromWorkspace  VariableName=testSig_EngPrt_trqLim  Interpolate=off  OutputAfterFinalValue=Holding final value
  spec_EngReq_trqInrLimSmk : FromWorkspace  VariableName=testSig_EngReq_trqInrLimSmk  Interpolate=off  OutputAfterFinalValue=Holding final value
  spec_EngReq_trqLim : FromWorkspace  VariableName=testSig_EngReq_trqLim  Interpolate=off  OutputAfterFinalValue=Holding final value
  spec_Epm_nEng : FromWorkspace  VariableName=testSig_Epm_nEng  Interpolate=off  OutputAfterFinalValue=Holding final value
  spec_GlbDa_stTrqDem : FromWorkspace  VariableName=testSig_GlbDa_stTrqDem  Interpolate=off  OutputAfterFinalValue=Holding final value
  spec_PFltLd_resFlw : FromWorkspace  VariableName=testSig_PFltLd_resFlw  Interpolate=off  OutputAfterFinalValue=Holding final value
  spec_TCPrt_trqInrBstPrtLim : FromWorkspace  VariableName=testSig_TCPrt_trqInrBstPrtLim  Interpolate=off  OutputAfterFinalValue=Holding final value
  spec_Tra_trqDblClthEngMax : FromWorkspace  VariableName=testSig_Tra_trqDblClthEngMax  Interpolate=off  OutputAfterFinalValue=Holding final value
  testSignals : Outport
  wires:
  BC/1 -> testSignals/1
  spec_Epm_nEng/1 -> BC/1  "testSig_Epm_nEng"
  spec_Tra_trqDblClthEngMax/1 -> BC/2  "testSig_Tra_trqDblClthEngMax"
  spec_TCPrt_trqInrBstPrtLim/1 -> BC/3  "testSig_TCPrt_trqInrBstPrtLim"
  spec_EngReq_trqLim/1 -> BC/4  "testSig_EngReq_trqLim"
  spec_GlbDa_stTrqDem/1 -> BC/5  "testSig_GlbDa_stTrqDem"
  spec_EngReq_trqInrLimSmk/1 -> BC/6  "testSig_EngReq_trqInrLimSmk"
  spec_EngPrt_trqLim/1 -> BC/7  "testSig_EngPrt_trqLim"
  spec_DSM_bEngDemTrqLimErr1/1 -> BC/8  "testSig_DSM_bEngDemTrqLimErr1"
  spec_DSM_bEngDemTrqLimErr2/1 -> BC/9  "testSig_DSM_bEngDemTrqLimErr2"
  spec_DSM_bEngDemTrqLimErr3/1 -> BC/10  "testSig_DSM_bEngDemTrqLimErr3"
  spec_DSM_bEngDemTrqLimErr4/1 -> BC/11  "testSig_DSM_bEngDemTrqLimErr4"
  spec_ASMod_dvolPFltEG/1 -> BC/12  "testSig_ASMod_dvolPFltEG"
  spec_PFltLd_resFlw/1 -> BC/13  "testSig_PFltLd_resFlw"
  spec_CoETS_trqNTCLim/1 -> BC/14  "testSig_CoETS_trqNTCLim"
  spec_CoVeh_trqPrfmLimDes/1 -> BC/15  "testSig_CoVeh_trqPrfmLimDes"
  spec_EngDem_trqLimErr/1 -> BC/16  "testSig_EngDem_trqLimErr"
  spec_EngDem_trqLimPDiff/1 -> BC/17  "testSig_EngDem_trqLimPDiff"
  spec_EngDem_trqInrLim/1 -> BC/18  "testSig_EngDem_trqInrLim"
  spec_EngDem_stErr_mp/1 -> BC/19  "testSig_EngDem_stErr_mp"
  spec_EngDem_facAdj/1 -> BC/20  "testSig_EngDem_facAdj"
  spec_EngDem_trqInrLimLead/1 -> BC/21  "testSig_EngDem_trqInrLimLead"
  spec_EngDem_trqInrLimSlow/1 -> BC/22  "testSig_EngDem_trqInrLimSlow"

== system TST_EngDem_TrqLimCoord/simulationInput/testSignals_R003 ==
  BC : BusCreator  Inputs=22
  spec_ASMod_dvolPFltEG : FromWorkspace  VariableName=testSig_ASMod_dvolPFltEG  Interpolate=off  OutputAfterFinalValue=Holding final value
  spec_CoETS_trqNTCLim : FromWorkspace  VariableName=testSig_CoETS_trqNTCLim  Interpolate=off  OutputAfterFinalValue=Holding final value
  spec_CoVeh_trqPrfmLimDes : FromWorkspace  VariableName=testSig_CoVeh_trqPrfmLimDes  Interpolate=off  OutputAfterFinalValue=Holding final value
  spec_DSM_bEngDemTrqLimErr1 : FromWorkspace  VariableName=testSig_DSM_bEngDemTrqLimErr1  Interpolate=off  OutputAfterFinalValue=Holding final value
  spec_DSM_bEngDemTrqLimErr2 : FromWorkspace  VariableName=testSig_DSM_bEngDemTrqLimErr2  Interpolate=off  OutputAfterFinalValue=Holding final value
  spec_DSM_bEngDemTrqLimErr3 : FromWorkspace  VariableName=testSig_DSM_bEngDemTrqLimErr3  Interpolate=off  OutputAfterFinalValue=Holding final value
  spec_DSM_bEngDemTrqLimErr4 : FromWorkspace  VariableName=testSig_DSM_bEngDemTrqLimErr4  Interpolate=off  OutputAfterFinalValue=Holding final value
  spec_EngDem_facAdj : FromWorkspace  VariableName=testSig_EngDem_facAdj  Interpolate=off  OutputAfterFinalValue=Holding final value
  spec_EngDem_stErr_mp : FromWorkspace  VariableName=testSig_EngDem_stErr_mp  Interpolate=off  OutputAfterFinalValue=Holding final value
  spec_EngDem_trqInrLim : FromWorkspace  VariableName=testSig_EngDem_trqInrLim  Interpolate=off  OutputAfterFinalValue=Holding final value
  spec_EngDem_trqInrLimLead : FromWorkspace  VariableName=testSig_EngDem_trqInrLimLead  Interpolate=off  OutputAfterFinalValue=Holding final value
  spec_EngDem_trqInrLimSlow : FromWorkspace  VariableName=testSig_EngDem_trqInrLimSlow  Interpolate=off  OutputAfterFinalValue=Holding final value
  spec_EngDem_trqLimErr : FromWorkspace  VariableName=testSig_EngDem_trqLimErr  Interpolate=off  OutputAfterFinalValue=Holding final value
  spec_EngDem_trqLimPDiff : FromWorkspace  VariableName=testSig_EngDem_trqLimPDiff  Interpolate=off  OutputAfterFinalValue=Holding final value
  spec_EngPrt_trqLim : FromWorkspace  VariableName=testSig_EngPrt_trqLim  Interpolate=off  OutputAfterFinalValue=Holding final value
  spec_EngReq_trqInrLimSmk : FromWorkspace  VariableName=testSig_EngReq_trqInrLimSmk  Interpolate=off  OutputAfterFinalValue=Holding final value
  spec_EngReq_trqLim : FromWorkspace  VariableName=testSig_EngReq_trqLim  Interpolate=off  OutputAfterFinalValue=Holding final value
  spec_Epm_nEng : FromWorkspace  VariableName=testSig_Epm_nEng  Interpolate=off  OutputAfterFinalValue=Holding final value
  spec_GlbDa_stTrqDem : FromWorkspace  VariableName=testSig_GlbDa_stTrqDem  Interpolate=off  OutputAfterFinalValue=Holding final value
  spec_PFltLd_resFlw : FromWorkspace  VariableName=testSig_PFltLd_resFlw  Interpolate=off  OutputAfterFinalValue=Holding final value
  spec_TCPrt_trqInrBstPrtLim : FromWorkspace  VariableName=testSig_TCPrt_trqInrBstPrtLim  Interpolate=off  OutputAfterFinalValue=Holding final value
  spec_Tra_trqDblClthEngMax : FromWorkspace  VariableName=testSig_Tra_trqDblClthEngMax  Interpolate=off  OutputAfterFinalValue=Holding final value
  testSignals : Outport
  wires:
  BC/1 -> testSignals/1
  spec_Epm_nEng/1 -> BC/1  "testSig_Epm_nEng"
  spec_Tra_trqDblClthEngMax/1 -> BC/2  "testSig_Tra_trqDblClthEngMax"
  spec_TCPrt_trqInrBstPrtLim/1 -> BC/3  "testSig_TCPrt_trqInrBstPrtLim"
  spec_EngReq_trqLim/1 -> BC/4  "testSig_EngReq_trqLim"
  spec_GlbDa_stTrqDem/1 -> BC/5  "testSig_GlbDa_stTrqDem"
  spec_EngReq_trqInrLimSmk/1 -> BC/6  "testSig_EngReq_trqInrLimSmk"
  spec_EngPrt_trqLim/1 -> BC/7  "testSig_EngPrt_trqLim"
  spec_DSM_bEngDemTrqLimErr1/1 -> BC/8  "testSig_DSM_bEngDemTrqLimErr1"
  spec_DSM_bEngDemTrqLimErr2/1 -> BC/9  "testSig_DSM_bEngDemTrqLimErr2"
  spec_DSM_bEngDemTrqLimErr3/1 -> BC/10  "testSig_DSM_bEngDemTrqLimErr3"
  spec_DSM_bEngDemTrqLimErr4/1 -> BC/11  "testSig_DSM_bEngDemTrqLimErr4"
  spec_ASMod_dvolPFltEG/1 -> BC/12  "testSig_ASMod_dvolPFltEG"
  spec_PFltLd_resFlw/1 -> BC/13  "testSig_PFltLd_resFlw"
  spec_CoETS_trqNTCLim/1 -> BC/14  "testSig_CoETS_trqNTCLim"
  spec_CoVeh_trqPrfmLimDes/1 -> BC/15  "testSig_CoVeh_trqPrfmLimDes"
  spec_EngDem_trqLimErr/1 -> BC/16  "testSig_EngDem_trqLimErr"
  spec_EngDem_trqLimPDiff/1 -> BC/17  "testSig_EngDem_trqLimPDiff"
  spec_EngDem_trqInrLim/1 -> BC/18  "testSig_EngDem_trqInrLim"
  spec_EngDem_stErr_mp/1 -> BC/19  "testSig_EngDem_stErr_mp"
  spec_EngDem_facAdj/1 -> BC/20  "testSig_EngDem_facAdj"
  spec_EngDem_trqInrLimLead/1 -> BC/21  "testSig_EngDem_trqInrLimLead"
  spec_EngDem_trqInrLimSlow/1 -> BC/22  "testSig_EngDem_trqInrLimSlow"
